simulink model "StopWatchStatechart"  (Simulink 10.1)
settings: Solver=FixedStepAuto  StartTime=0.0  StopTime=1000.0  FixedStep=1e-3  RelTol=1e-3
settings Model: Creator=Lukas Bilal  LastModifiedBy=Lukas Bilal  EnablePacing=on
settings DataIOCC: SaveFormat=Dataset  ReturnWorkspaceOutputs=on
settings OptimizationCC: LifeSpan=auto
settings DebuggingCC: UnderspecifiedInitializationDetection=Simplified  MergeDetectMultiDrivingBlocksExec=error  SFUnexpectedBacktrackingDiag=error  SFNoUnconditionalDefaultTransitionDiag=error  SFExecutionAtInitializationDiag=warning  ArithmeticOperatorsInVariantConditions=error
settings HardwareCC: ProdBitPerPointer=64  ProdBitPerSizeT=64  ProdBitPerPtrDiffT=64  ProdLargestAtomicFloat=Float  ProdIntDivRoundTo=Zero  ProdEndianess=LittleEndian  ProdWordSize=64  ProdHWDeviceType=Intel->x86-64 (Windows64)
settings ModelReferenceCC: PropagateSignalLabelsOutOfModel=on
settings SFSimCC: SimUseLocalCustomCode=on  CustomCodeUndefinedFunction=FilterOut
settings RTWCC: RTWUseLocalCustomCode=on
settings CodeAppCC: StateflowObjectComments=off
settings GRTTargetCC: TargetLangStandard=C99 (ISO)  CombineOutputUpdateFcns=on  GRTInterface=off
settings ConfigComp: CovMetricSettings=dwe  CovHtmlReporting=off  CovSaveCumulativeToWorkspaceVar=off  CovSaveSingleToWorkspaceVar=off  CovExternalEMLEnable=on

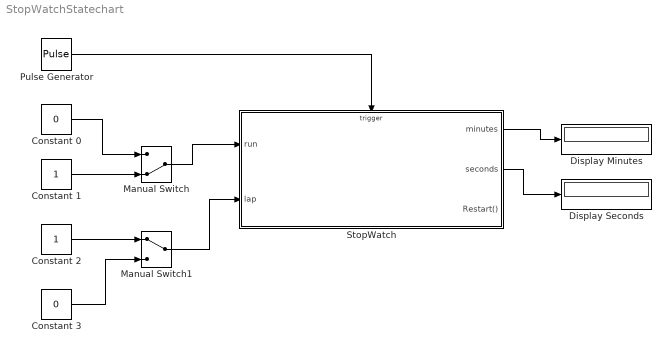
== system StopWatchStatechart ==
  Constant 0 : Constant  Value=0  OutDataTypeStr=boolean
  Constant 1 : Constant  OutDataTypeStr=boolean
  Constant 2 : Constant  OutDataTypeStr=boolean
  Constant 3 : Constant  Value=0  OutDataTypeStr=boolean
  Display Minutes : Display
  Display Seconds : Display
  Manual Switch : ManualSwitch  CurrentSetting=0
  Manual Switch1 : ManualSwitch
  "Pulse Generator " : DiscretePulseGenerator  PulseType=Time based  Period=1  PulseWidth=5
  StopWatch : Stateflow chart  TreatAsAtomicUnit=on
  wires:
  "Pulse Generator "/1 -> StopWatch/Trigger
  Constant 0/1 -> Manual Switch/1
  Constant 1/1 -> Manual Switch/2
  Manual Switch/1 -> StopWatch/1(run)
  StopWatch/1(minutes) -> Display Minutes/1
  StopWatch/2(seconds) -> Display Seconds/1
  Constant 2/1 -> Manual Switch1/1
  Constant 3/1 -> Manual Switch1/2
  Manual Switch1/1 -> StopWatch/2(lap)

== stateflow chart StopWatch ==
  settings: executeAtInitialization=1
  state Stopped
    state Recall
    state Store
    state Restart
    (default) -> Store
    Store -> Restart [order 2] : Restart
    Recall -> Store [order 1] : storeRecall /
        | {
        |   minutes_intern = 0;
        |   seconds_intern = 0;
        |   seconds_stored = 0;
        |   minutes_stored = 0;
        | }
    Store -> Recall [order 1] : storeRecall /
        | {
        |   minutes_intern = minutes_stored;
        |   seconds_intern = seconds_stored;
        | }
    Restart -> Restart : {
        |   minutes_intern = 0;
        |   seconds_intern = 0;
        |   seconds_stored = 0;
        |   minutes_stored = 0;
        |   run = 1;
        | }
    Recall -> Restart [order 2] : Restart
  state Started
    state Lab [parallel]
      settings: executionOrder=1
      state lab
      (default) -> lab
      lab -> lab : [lap] /
          | {
          |   seconds = seconds_intern;
          |   minutes = minutes_intern;
          | }
    state Clock [parallel]
      settings: executionOrder=2
      state Clock
      (default) -> Started.Clock.Clock
      Started.Clock.Clock -> Started.Clock.Clock [order 1] : clk [seconds_intern < 59] /
          | {
          |   seconds_intern = seconds_intern + 1;
          | }
      Started.Clock.Clock -> Started.Clock.Clock [order 2] : clk [seconds_intern == 59]
          | {
          |   minutes_intern = minutes_intern + 1;
          |   seconds_intern = 0;
          | }
    state store_recall [parallel]
      settings: executionOrder=3
      state store
      state recall
      (default) -> store
      recall -> store : storeRecall /
          | {
          |   seconds_stored = seconds_intern;
          |   minutes_stored = minutes_intern;
          | }
      store -> recall : storeRecall /
          | {
          |   seconds_intern = seconds_stored;
          |   minutes_intern = minutes_stored;
          | }
  (default) -> Stopped
  Stopped -> Started : [run]
  Started -> Stopped : [~run]
  data: minutes output uint32; seconds output uint8; run input boolean; lap input boolean; minutes_intern local uint32; seconds_intern local uint8; seconds_stored local double; minutes_stored local double
  events: clk input RISING_EDGE_EVENT; storeRecall input EITHER_EDGE_EVENT; Restart output FUNCTION_CALL_EVENT
